simulink model "task_2_1a"  (R2021b)
settings: Solver=FixedStepAuto  StartTime=0.0  StopTime=5  FixedStep=0.01  RelTol=1e-3
settings Model: Creator=osini  LastModifiedBy=osini

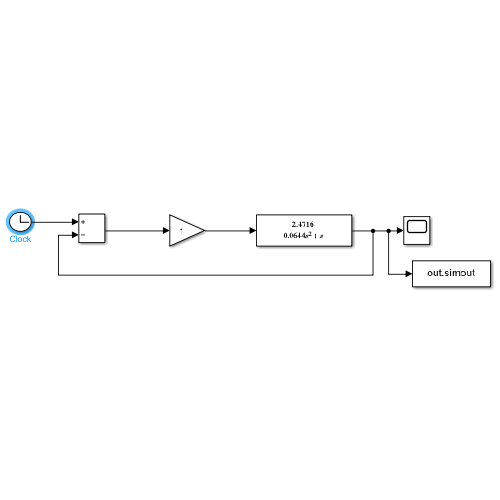
[thumbnail: Simulink's stored preview of the top-level diagram]
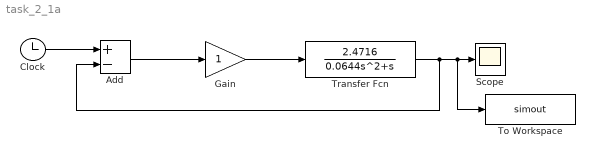
== system task_2_1a ==
  Add : Sum  Inputs=+-
  Clock : Clock
  Gain : Gain
  Scope : Scope
  To Workspace : ToWorkspace  VariableName=simout  SaveFormat=Timeseries  SampleTime=-1
  Transfer Fcn : TransferFcn  Numerator=[2.4716]  Denominator=[0.0644 1 0]
  wires:
  Add/1 -> Gain/1
  Gain/1 -> Transfer Fcn/1
  Transfer Fcn/1 -> Add/2, To Workspace/1, Scope/1
  Clock/1 -> Add/1
